simulink model "cic_dec3_4inputs_model"  (Simulink 7.4)
settings: Solver=ode45  StartTime=0.0  StopTime=10.0  RelTol=1e-3
libraries: xbsIndex_r4 x76
settings Model: Creator=chenhong  LastModifiedBy=chenhong

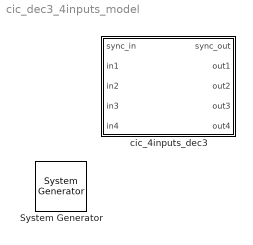
== system cic_dec3_4inputs_model ==
  " System Generator" : xbsIndex_r4/ System Generator  Tag=genX  SystemSampleTime=-1  xilinxfamily=Virtex6  part=xc6vsx315t  speed=-3  package=ff1156  synthesis_tool=XST  clock_wrapper=Clock Enables  directory=./netlist  testbench=off  simulink_period=1  sysclk_period=10  dcm_input_clock_period=10  incr_netlist=off  trim_vbits=Everywhere in SubSystem  dbl_ovrd=According to Block Masks  core_generation=According to Block Masks  run_coregen=off  deprecated_control=off  eval_field=0  block_type=sysgen
      settings: block_version=11.4
  cic_4inputs_dec3 : Subsystem

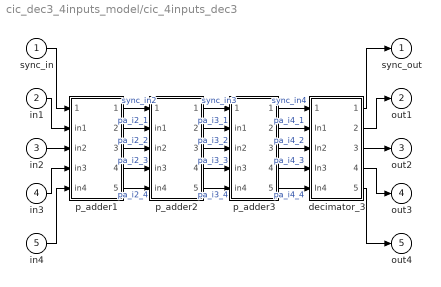
== system cic_dec3_4inputs_model/cic_4inputs_dec3 ==
  sync_in : Inport
  in1 : Inport  Port=2
  in2 : Inport  Port=3
  in3 : Inport  Port=4
  in4 : Inport  Port=5
  decimator_3 : Subsystem
  p_adder1 : Subsystem
  p_adder2 : Subsystem
  p_adder3 : Subsystem
  sync_out : Outport
  out1 : Outport  Port=2
  out2 : Outport  Port=3
  out3 : Outport  Port=4
  out4 : Outport  Port=5
  wires:
  decimator_3/4(Out3) -> out3/1
  decimator_3/2(Out1) -> out1/1
  p_adder3/5(out4) -> decimator_3/5(In4)  "pa_i4_4"
  p_adder3/3(out2) -> decimator_3/3(In2)  "pa_i4_2"
  p_adder3/1(sync_out) -> decimator_3/1(sync_in)  "sync_in4"
  p_adder2/5(out4) -> p_adder3/5(in4)  "pa_i3_4"
  p_adder2/3(out2) -> p_adder3/3(in2)  "pa_i3_2"
  p_adder2/1(sync_out) -> p_adder3/1(sync_in)  "sync_in3"
  p_adder1/5(out4) -> p_adder2/5(in4)  "pa_i2_4"
  p_adder1/3(out2) -> p_adder2/3(in2)  "pa_i2_2"
  p_adder1/1(sync_out) -> p_adder2/1(sync_in)  "sync_in2"
  in4/1 -> p_adder1/5(in4)
  in2/1 -> p_adder1/3(in2)
  sync_in/1 -> p_adder1/1(sync_in)
  in1/1 -> p_adder1/2(in1)
  in3/1 -> p_adder1/4(in3)
  p_adder1/2(out1) -> p_adder2/2(in1)  "pa_i2_1"
  p_adder1/4(out3) -> p_adder2/4(in3)  "pa_i2_3"
  p_adder2/2(out1) -> p_adder3/2(in1)  "pa_i3_1"
  p_adder2/4(out3) -> p_adder3/4(in3)  "pa_i3_3"
  p_adder3/2(out1) -> decimator_3/2(In1)  "pa_i4_1"
  p_adder3/4(out3) -> decimator_3/4(In3)  "pa_i4_3"
  decimator_3/1(sync_out) -> sync_out/1
  decimator_3/3(Out2) -> out2/1
  decimator_3/5(Out4) -> out4/1

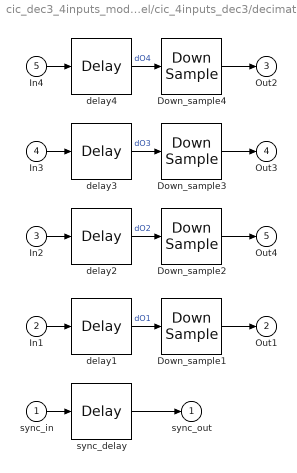
== system cic_dec3_4inputs_model/cic_4inputs_dec3/decimator_3 ==
  sync_in : Inport
  In1 : Inport  Port=2
  In2 : Inport  Port=3
  In3 : Inport  Port=4
  In4 : Inport  Port=5
  Down_sample{1..4} (4 alike) : xbsIndex_r4/Down Sample  sample_ratio=3  sample_phase="Last Value of Frame  (most efficient)"  en=off  latency=1  dbl_ovrd=off  block_type=dsamp
      settings: block_version=11.4
  delay1 : xbsIndex_r4/Delay  en=off  latency=2  dbl_ovrd=off  reg_retiming=off  block_type=delay
      settings: block_version=11.4
  delay2 : xbsIndex_r4/Delay  en=off  latency=0  dbl_ovrd=off  reg_retiming=off  block_type=delay
      settings: block_version=11.4
  delay3 : xbsIndex_r4/Delay  en=off  latency=1  dbl_ovrd=off  reg_retiming=off  block_type=delay
      settings: block_version=11.4
  delay4 : xbsIndex_r4/Delay  en=off  latency=2  dbl_ovrd=off  reg_retiming=off  block_type=delay
      settings: block_version=11.4
  sync_delay : xbsIndex_r4/Delay  en=off  latency=1  dbl_ovrd=off  reg_retiming=off  block_type=delay
      settings: block_version=11.4
  sync_out : Outport
  Out1 : Outport  Port=2
  Out2 : Outport  Port=3
  Out3 : Outport  Port=4
  Out4 : Outport  Port=5
  wires:
  sync_in/1 -> sync_delay/1
  Down_sample4/1 -> Out2/1
  delay3/1 -> Down_sample3/1  "dO3"
  In3/1 -> delay3/1
  Down_sample2/1 -> Out4/1
  delay1/1 -> Down_sample1/1  "dO1"
  In1/1 -> delay1/1
  Down_sample1/1 -> Out1/1
  In2/1 -> delay2/1
  delay2/1 -> Down_sample2/1  "dO2"
  Down_sample3/1 -> Out3/1
  In4/1 -> delay4/1
  delay4/1 -> Down_sample4/1  "dO4"
  sync_delay/1 -> sync_out/1

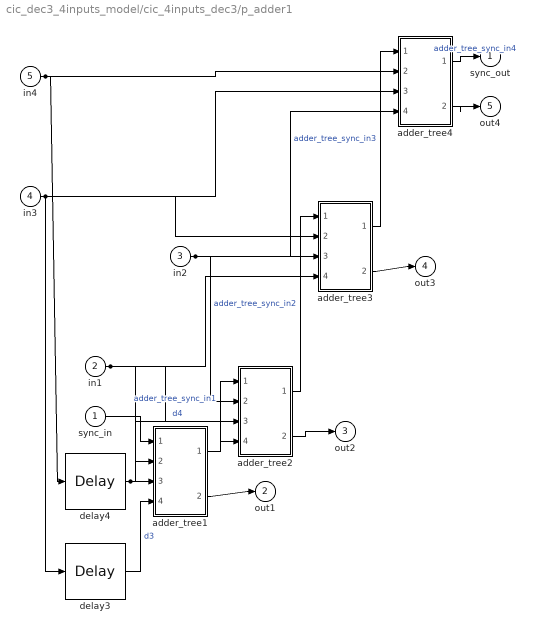
== system cic_dec3_4inputs_model/cic_4inputs_dec3/p_adder1 ==
  sync_in : Inport
  in1 : Inport  Port=2
  in2 : Inport  Port=3
  in3 : Inport  Port=4
  in4 : Inport  Port=5
  adder_tree1 : Subsystem
  adder_tree2 : Subsystem
  adder_tree3 : Subsystem
  adder_tree4 : Subsystem
  delay3 : xbsIndex_r4/Delay  en=off  latency=1  dbl_ovrd=off  reg_retiming=off  block_type=delay
      settings: block_version=11.4
  delay4 : xbsIndex_r4/Delay  en=off  latency=1  dbl_ovrd=off  reg_retiming=off  block_type=delay
      settings: block_version=11.4
  sync_out : Outport
  out1 : Outport  Port=2
  out2 : Outport  Port=3
  out3 : Outport  Port=4
  out4 : Outport  Port=5
  wires:
  in1/1 -> adder_tree2/3(din_2), adder_tree1/2(din_1), adder_tree3/4(din_3)
  delay4/1 -> adder_tree1/3(din_2), adder_tree2/4(din_3)  "d4"
  in3/1 -> adder_tree4/3(din_2), delay3/1, adder_tree3/2(din_1)
  in2/1 -> adder_tree3/3(din_2), adder_tree2/2(din_1), adder_tree4/4(din_3)
  in4/1 -> delay4/1, adder_tree4/2(din_1)
  adder_tree4/1(sync_out) -> sync_out/1  "adder_tree_sync_in4"
  adder_tree4/2(dout) -> out4/1
  adder_tree3/1(sync_out) -> adder_tree4/1(sync)  "adder_tree_sync_in3"
  adder_tree3/2(dout) -> out3/1
  adder_tree2/1(sync_out) -> adder_tree3/1(sync)  "adder_tree_sync_in2"
  adder_tree2/2(dout) -> out2/1
  adder_tree1/1(sync_out) -> adder_tree2/1(sync)  "adder_tree_sync_in1"
  adder_tree1/2(dout) -> out1/1
  sync_in/1 -> adder_tree1/1(sync)
  delay3/1 -> adder_tree1/4(din_3)  "d3"

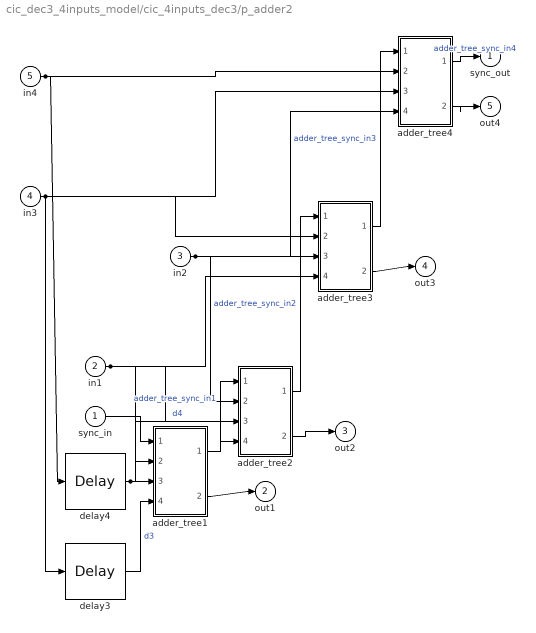
== system cic_dec3_4inputs_model/cic_4inputs_dec3/p_adder2 ==
  sync_in : Inport
  in1 : Inport  Port=2
  in2 : Inport  Port=3
  in3 : Inport  Port=4
  in4 : Inport  Port=5
  adder_tree1 : Subsystem
  adder_tree2 : Subsystem
  adder_tree3 : Subsystem
  adder_tree4 : Subsystem
  delay3 : xbsIndex_r4/Delay  en=off  latency=1  dbl_ovrd=off  reg_retiming=off  block_type=delay
      settings: block_version=11.4
  delay4 : xbsIndex_r4/Delay  en=off  latency=1  dbl_ovrd=off  reg_retiming=off  block_type=delay
      settings: block_version=11.4
  sync_out : Outport
  out1 : Outport  Port=2
  out2 : Outport  Port=3
  out3 : Outport  Port=4
  out4 : Outport  Port=5
  wires:
  in1/1 -> adder_tree2/3(din_2), adder_tree1/2(din_1), adder_tree3/4(din_3)
  delay4/1 -> adder_tree1/3(din_2), adder_tree2/4(din_3)  "d4"
  in3/1 -> adder_tree4/3(din_2), delay3/1, adder_tree3/2(din_1)
  in2/1 -> adder_tree3/3(din_2), adder_tree2/2(din_1), adder_tree4/4(din_3)
  in4/1 -> delay4/1, adder_tree4/2(din_1)
  adder_tree4/1(sync_out) -> sync_out/1  "adder_tree_sync_in4"
  adder_tree4/2(dout) -> out4/1
  adder_tree3/1(sync_out) -> adder_tree4/1(sync)  "adder_tree_sync_in3"
  adder_tree3/2(dout) -> out3/1
  adder_tree2/1(sync_out) -> adder_tree3/1(sync)  "adder_tree_sync_in2"
  adder_tree2/2(dout) -> out2/1
  adder_tree1/1(sync_out) -> adder_tree2/1(sync)  "adder_tree_sync_in1"
  adder_tree1/2(dout) -> out1/1
  sync_in/1 -> adder_tree1/1(sync)
  delay3/1 -> adder_tree1/4(din_3)  "d3"

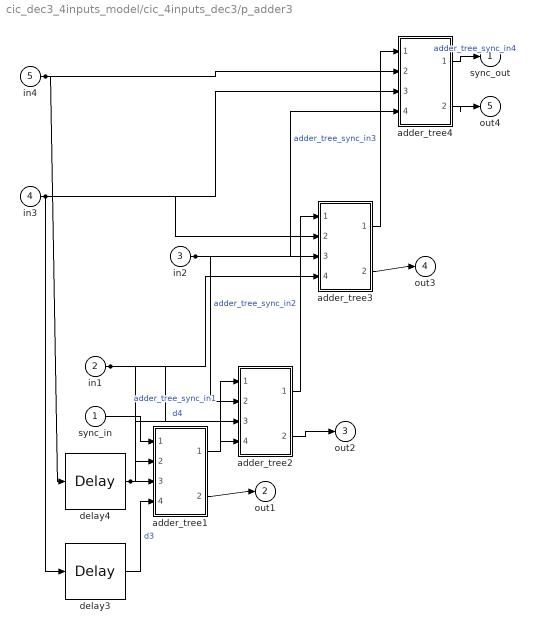
== system cic_dec3_4inputs_model/cic_4inputs_dec3/p_adder3 ==
  sync_in : Inport
  in1 : Inport  Port=2
  in2 : Inport  Port=3
  in3 : Inport  Port=4
  in4 : Inport  Port=5
  adder_tree1 : Subsystem
  adder_tree2 : Subsystem
  adder_tree3 : Subsystem
  adder_tree4 : Subsystem
  delay3 : xbsIndex_r4/Delay  en=off  latency=1  dbl_ovrd=off  reg_retiming=off  block_type=delay
      settings: block_version=11.4
  delay4 : xbsIndex_r4/Delay  en=off  latency=1  dbl_ovrd=off  reg_retiming=off  block_type=delay
      settings: block_version=11.4
  sync_out : Outport
  out1 : Outport  Port=2
  out2 : Outport  Port=3
  out3 : Outport  Port=4
  out4 : Outport  Port=5
  wires:
  in1/1 -> adder_tree2/3(din_2), adder_tree1/2(din_1), adder_tree3/4(din_3)
  delay4/1 -> adder_tree1/3(din_2), adder_tree2/4(din_3)  "d4"
  in3/1 -> adder_tree4/3(din_2), delay3/1, adder_tree3/2(din_1)
  in2/1 -> adder_tree3/3(din_2), adder_tree2/2(din_1), adder_tree4/4(din_3)
  in4/1 -> delay4/1, adder_tree4/2(din_1)
  adder_tree4/1(sync_out) -> sync_out/1  "adder_tree_sync_in4"
  adder_tree4/2(dout) -> out4/1
  adder_tree3/1(sync_out) -> adder_tree4/1(sync)  "adder_tree_sync_in3"
  adder_tree3/2(dout) -> out3/1
  adder_tree2/1(sync_out) -> adder_tree3/1(sync)  "adder_tree_sync_in2"
  adder_tree2/2(dout) -> out2/1
  adder_tree1/1(sync_out) -> adder_tree2/1(sync)  "adder_tree_sync_in1"
  adder_tree1/2(dout) -> out1/1
  sync_in/1 -> adder_tree1/1(sync)
  delay3/1 -> adder_tree1/4(din_3)  "d3"

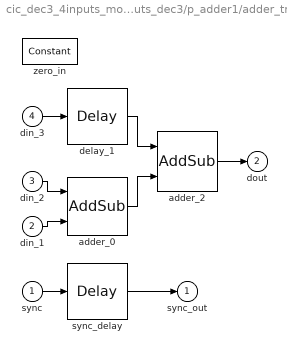
== system cic_dec3_4inputs_model/cic_4inputs_dec3/p_adder1/adder_tree1 ==
  sync : Inport
  din_1 : Inport  Port=2
  din_2 : Inport  Port=3
  din_3 : Inport  Port=4
  adder_0 : xbsIndex_r4/AddSub  mode=Addition  use_carryin=off  use_carryout=off  en=off  latency=1  precision=Full  arith_type=Unsigned  n_bits=16  bin_pt=14  quantization="Round  (unbiased: +/- Inf)"  overflow=Saturate  dbl_ovrd=off  use_behavioral_HDL=on  hw_selection=Fabric  pipelined=off  block_type=addsub
  adder_2 : xbsIndex_r4/AddSub  mode=Addition  use_carryin=off  use_carryout=off  en=off  latency=1  precision=Full  arith_type=Unsigned  n_bits=16  bin_pt=14  quantization="Round  (unbiased: +/- Inf)"  overflow=Saturate  dbl_ovrd=off  use_behavioral_HDL=on  hw_selection=Fabric  pipelined=off  block_type=addsub
  delay_1 : xbsIndex_r4/Delay  en=off  latency=1  dbl_ovrd=off  reg_retiming=off  block_type=delay
      settings: block_version=11.4
  sync_delay : xbsIndex_r4/Delay  en=off  latency=2  dbl_ovrd=off  reg_retiming=off  block_type=delay
      settings: block_version=11.4
  zero_in : xbsIndex_r4/Constant  arith_type=Unsigned  const=0  n_bits=18  bin_pt=17  explicit_period=off  period=1  equ=P=C  opselect=C  inp2=PCIN>>17  opr=+  inp1=P  carry=CIN  dbl_ovrd=off  block_type=constant
      settings: block_version=11.4
  sync_out : Outport
  dout : Outport  Port=2
  wires:
  adder_0/1 -> adder_2/2
  din_2/1 -> adder_0/1
  sync/1 -> sync_delay/1
  sync_delay/1 -> sync_out/1
  din_1/1 -> adder_0/2
  din_3/1 -> delay_1/1
  delay_1/1 -> adder_2/1
  adder_2/1 -> dout/1

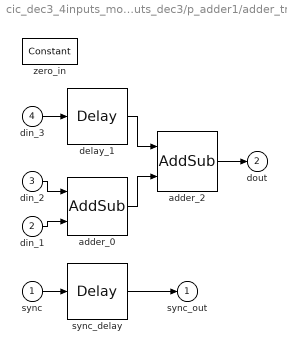
== system cic_dec3_4inputs_model/cic_4inputs_dec3/p_adder1/adder_tree2 ==
  sync : Inport
  din_1 : Inport  Port=2
  din_2 : Inport  Port=3
  din_3 : Inport  Port=4
  adder_0 : xbsIndex_r4/AddSub  mode=Addition  use_carryin=off  use_carryout=off  en=off  latency=1  precision=Full  arith_type=Unsigned  n_bits=16  bin_pt=14  quantization="Round  (unbiased: +/- Inf)"  overflow=Saturate  dbl_ovrd=off  use_behavioral_HDL=on  hw_selection=Fabric  pipelined=off  block_type=addsub
  adder_2 : xbsIndex_r4/AddSub  mode=Addition  use_carryin=off  use_carryout=off  en=off  latency=1  precision=Full  arith_type=Unsigned  n_bits=16  bin_pt=14  quantization="Round  (unbiased: +/- Inf)"  overflow=Saturate  dbl_ovrd=off  use_behavioral_HDL=on  hw_selection=Fabric  pipelined=off  block_type=addsub
  delay_1 : xbsIndex_r4/Delay  en=off  latency=1  dbl_ovrd=off  reg_retiming=off  block_type=delay
      settings: block_version=11.4
  sync_delay : xbsIndex_r4/Delay  en=off  latency=2  dbl_ovrd=off  reg_retiming=off  block_type=delay
      settings: block_version=11.4
  zero_in : xbsIndex_r4/Constant  arith_type=Unsigned  const=0  n_bits=18  bin_pt=17  explicit_period=off  period=1  equ=P=C  opselect=C  inp2=PCIN>>17  opr=+  inp1=P  carry=CIN  dbl_ovrd=off  block_type=constant
      settings: block_version=11.4
  sync_out : Outport
  dout : Outport  Port=2
  wires:
  adder_0/1 -> adder_2/2
  din_2/1 -> adder_0/1
  sync/1 -> sync_delay/1
  sync_delay/1 -> sync_out/1
  din_1/1 -> adder_0/2
  din_3/1 -> delay_1/1
  delay_1/1 -> adder_2/1
  adder_2/1 -> dout/1

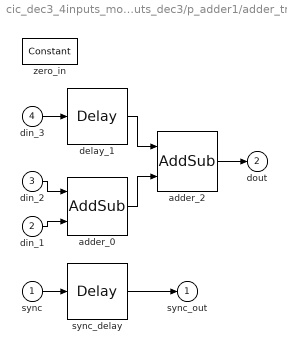
== system cic_dec3_4inputs_model/cic_4inputs_dec3/p_adder1/adder_tree3 ==
  sync : Inport
  din_1 : Inport  Port=2
  din_2 : Inport  Port=3
  din_3 : Inport  Port=4
  adder_0 : xbsIndex_r4/AddSub  mode=Addition  use_carryin=off  use_carryout=off  en=off  latency=1  precision=Full  arith_type=Unsigned  n_bits=16  bin_pt=14  quantization="Round  (unbiased: +/- Inf)"  overflow=Saturate  dbl_ovrd=off  use_behavioral_HDL=on  hw_selection=Fabric  pipelined=off  block_type=addsub
  adder_2 : xbsIndex_r4/AddSub  mode=Addition  use_carryin=off  use_carryout=off  en=off  latency=1  precision=Full  arith_type=Unsigned  n_bits=16  bin_pt=14  quantization="Round  (unbiased: +/- Inf)"  overflow=Saturate  dbl_ovrd=off  use_behavioral_HDL=on  hw_selection=Fabric  pipelined=off  block_type=addsub
  delay_1 : xbsIndex_r4/Delay  en=off  latency=1  dbl_ovrd=off  reg_retiming=off  block_type=delay
      settings: block_version=11.4
  sync_delay : xbsIndex_r4/Delay  en=off  latency=2  dbl_ovrd=off  reg_retiming=off  block_type=delay
      settings: block_version=11.4
  zero_in : xbsIndex_r4/Constant  arith_type=Unsigned  const=0  n_bits=18  bin_pt=17  explicit_period=off  period=1  equ=P=C  opselect=C  inp2=PCIN>>17  opr=+  inp1=P  carry=CIN  dbl_ovrd=off  block_type=constant
      settings: block_version=11.4
  sync_out : Outport
  dout : Outport  Port=2
  wires:
  adder_0/1 -> adder_2/2
  din_2/1 -> adder_0/1
  sync/1 -> sync_delay/1
  sync_delay/1 -> sync_out/1
  din_1/1 -> adder_0/2
  din_3/1 -> delay_1/1
  delay_1/1 -> adder_2/1
  adder_2/1 -> dout/1

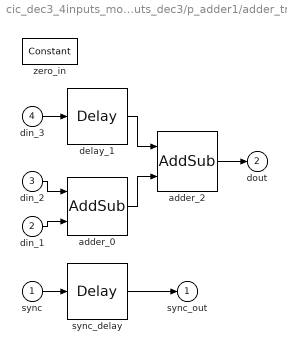
== system cic_dec3_4inputs_model/cic_4inputs_dec3/p_adder1/adder_tree4 ==
  sync : Inport
  din_1 : Inport  Port=2
  din_2 : Inport  Port=3
  din_3 : Inport  Port=4
  adder_0 : xbsIndex_r4/AddSub  mode=Addition  use_carryin=off  use_carryout=off  en=off  latency=1  precision=Full  arith_type=Unsigned  n_bits=16  bin_pt=14  quantization="Round  (unbiased: +/- Inf)"  overflow=Saturate  dbl_ovrd=off  use_behavioral_HDL=on  hw_selection=Fabric  pipelined=off  block_type=addsub
  adder_2 : xbsIndex_r4/AddSub  mode=Addition  use_carryin=off  use_carryout=off  en=off  latency=1  precision=Full  arith_type=Unsigned  n_bits=16  bin_pt=14  quantization="Round  (unbiased: +/- Inf)"  overflow=Saturate  dbl_ovrd=off  use_behavioral_HDL=on  hw_selection=Fabric  pipelined=off  block_type=addsub
  delay_1 : xbsIndex_r4/Delay  en=off  latency=1  dbl_ovrd=off  reg_retiming=off  block_type=delay
      settings: block_version=11.4
  sync_delay : xbsIndex_r4/Delay  en=off  latency=2  dbl_ovrd=off  reg_retiming=off  block_type=delay
      settings: block_version=11.4
  zero_in : xbsIndex_r4/Constant  arith_type=Unsigned  const=0  n_bits=18  bin_pt=17  explicit_period=off  period=1  equ=P=C  opselect=C  inp2=PCIN>>17  opr=+  inp1=P  carry=CIN  dbl_ovrd=off  block_type=constant
      settings: block_version=11.4
  sync_out : Outport
  dout : Outport  Port=2
  wires:
  adder_0/1 -> adder_2/2
  din_2/1 -> adder_0/1
  sync/1 -> sync_delay/1
  sync_delay/1 -> sync_out/1
  din_1/1 -> adder_0/2
  din_3/1 -> delay_1/1
  delay_1/1 -> adder_2/1
  adder_2/1 -> dout/1

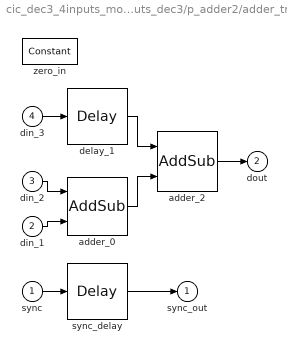
== system cic_dec3_4inputs_model/cic_4inputs_dec3/p_adder2/adder_tree1 ==
  sync : Inport
  din_1 : Inport  Port=2
  din_2 : Inport  Port=3
  din_3 : Inport  Port=4
  adder_0 : xbsIndex_r4/AddSub  mode=Addition  use_carryin=off  use_carryout=off  en=off  latency=1  precision=Full  arith_type=Unsigned  n_bits=16  bin_pt=14  quantization="Round  (unbiased: +/- Inf)"  overflow=Saturate  dbl_ovrd=off  use_behavioral_HDL=on  hw_selection=Fabric  pipelined=off  block_type=addsub
  adder_2 : xbsIndex_r4/AddSub  mode=Addition  use_carryin=off  use_carryout=off  en=off  latency=1  precision=Full  arith_type=Unsigned  n_bits=16  bin_pt=14  quantization="Round  (unbiased: +/- Inf)"  overflow=Saturate  dbl_ovrd=off  use_behavioral_HDL=on  hw_selection=Fabric  pipelined=off  block_type=addsub
  delay_1 : xbsIndex_r4/Delay  en=off  latency=1  dbl_ovrd=off  reg_retiming=off  block_type=delay
      settings: block_version=11.4
  sync_delay : xbsIndex_r4/Delay  en=off  latency=2  dbl_ovrd=off  reg_retiming=off  block_type=delay
      settings: block_version=11.4
  zero_in : xbsIndex_r4/Constant  arith_type=Unsigned  const=0  n_bits=18  bin_pt=17  explicit_period=off  period=1  equ=P=C  opselect=C  inp2=PCIN>>17  opr=+  inp1=P  carry=CIN  dbl_ovrd=off  block_type=constant
      settings: block_version=11.4
  sync_out : Outport
  dout : Outport  Port=2
  wires:
  adder_0/1 -> adder_2/2
  din_2/1 -> adder_0/1
  sync/1 -> sync_delay/1
  sync_delay/1 -> sync_out/1
  din_1/1 -> adder_0/2
  din_3/1 -> delay_1/1
  delay_1/1 -> adder_2/1
  adder_2/1 -> dout/1

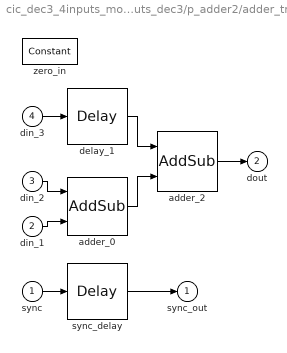
== system cic_dec3_4inputs_model/cic_4inputs_dec3/p_adder2/adder_tree2 ==
  sync : Inport
  din_1 : Inport  Port=2
  din_2 : Inport  Port=3
  din_3 : Inport  Port=4
  adder_0 : xbsIndex_r4/AddSub  mode=Addition  use_carryin=off  use_carryout=off  en=off  latency=1  precision=Full  arith_type=Unsigned  n_bits=16  bin_pt=14  quantization="Round  (unbiased: +/- Inf)"  overflow=Saturate  dbl_ovrd=off  use_behavioral_HDL=on  hw_selection=Fabric  pipelined=off  block_type=addsub
  adder_2 : xbsIndex_r4/AddSub  mode=Addition  use_carryin=off  use_carryout=off  en=off  latency=1  precision=Full  arith_type=Unsigned  n_bits=16  bin_pt=14  quantization="Round  (unbiased: +/- Inf)"  overflow=Saturate  dbl_ovrd=off  use_behavioral_HDL=on  hw_selection=Fabric  pipelined=off  block_type=addsub
  delay_1 : xbsIndex_r4/Delay  en=off  latency=1  dbl_ovrd=off  reg_retiming=off  block_type=delay
      settings: block_version=11.4
  sync_delay : xbsIndex_r4/Delay  en=off  latency=2  dbl_ovrd=off  reg_retiming=off  block_type=delay
      settings: block_version=11.4
  zero_in : xbsIndex_r4/Constant  arith_type=Unsigned  const=0  n_bits=18  bin_pt=17  explicit_period=off  period=1  equ=P=C  opselect=C  inp2=PCIN>>17  opr=+  inp1=P  carry=CIN  dbl_ovrd=off  block_type=constant
      settings: block_version=11.4
  sync_out : Outport
  dout : Outport  Port=2
  wires:
  adder_0/1 -> adder_2/2
  din_2/1 -> adder_0/1
  sync/1 -> sync_delay/1
  sync_delay/1 -> sync_out/1
  din_1/1 -> adder_0/2
  din_3/1 -> delay_1/1
  delay_1/1 -> adder_2/1
  adder_2/1 -> dout/1

== system cic_dec3_4inputs_model/cic_4inputs_dec3/p_adder2/adder_tree3 ==
  sync : Inport
  din_1 : Inport  Port=2
  din_2 : Inport  Port=3
  din_3 : Inport  Port=4
  adder_0 : xbsIndex_r4/AddSub  mode=Addition  use_carryin=off  use_carryout=off  en=off  latency=1  precision=Full  arith_type=Unsigned  n_bits=16  bin_pt=14  quantization="Round  (unbiased: +/- Inf)"  overflow=Saturate  dbl_ovrd=off  use_behavioral_HDL=on  hw_selection=Fabric  pipelined=off  block_type=addsub
  adder_2 : xbsIndex_r4/AddSub  mode=Addition  use_carryin=off  use_carryout=off  en=off  latency=1  precision=Full  arith_type=Unsigned  n_bits=16  bin_pt=14  quantization="Round  (unbiased: +/- Inf)"  overflow=Saturate  dbl_ovrd=off  use_behavioral_HDL=on  hw_selection=Fabric  pipelined=off  block_type=addsub
  delay_1 : xbsIndex_r4/Delay  en=off  latency=1  dbl_ovrd=off  reg_retiming=off  block_type=delay
      settings: block_version=11.4
  sync_delay : xbsIndex_r4/Delay  en=off  latency=2  dbl_ovrd=off  reg_retiming=off  block_type=delay
      settings: block_version=11.4
  zero_in : xbsIndex_r4/Constant  arith_type=Unsigned  const=0  n_bits=18  bin_pt=17  explicit_period=off  period=1  equ=P=C  opselect=C  inp2=PCIN>>17  opr=+  inp1=P  carry=CIN  dbl_ovrd=off  block_type=constant
      settings: block_version=11.4
  sync_out : Outport
  dout : Outport  Port=2
  wires:
  adder_0/1 -> adder_2/2
  din_2/1 -> adder_0/1
  sync/1 -> sync_delay/1
  sync_delay/1 -> sync_out/1
  din_1/1 -> adder_0/2
  din_3/1 -> delay_1/1
  delay_1/1 -> adder_2/1
  adder_2/1 -> dout/1

== system cic_dec3_4inputs_model/cic_4inputs_dec3/p_adder2/adder_tree4 ==
  sync : Inport
  din_1 : Inport  Port=2
  din_2 : Inport  Port=3
  din_3 : Inport  Port=4
  adder_0 : xbsIndex_r4/AddSub  mode=Addition  use_carryin=off  use_carryout=off  en=off  latency=1  precision=Full  arith_type=Unsigned  n_bits=16  bin_pt=14  quantization="Round  (unbiased: +/- Inf)"  overflow=Saturate  dbl_ovrd=off  use_behavioral_HDL=on  hw_selection=Fabric  pipelined=off  block_type=addsub
  adder_2 : xbsIndex_r4/AddSub  mode=Addition  use_carryin=off  use_carryout=off  en=off  latency=1  precision=Full  arith_type=Unsigned  n_bits=16  bin_pt=14  quantization="Round  (unbiased: +/- Inf)"  overflow=Saturate  dbl_ovrd=off  use_behavioral_HDL=on  hw_selection=Fabric  pipelined=off  block_type=addsub
  delay_1 : xbsIndex_r4/Delay  en=off  latency=1  dbl_ovrd=off  reg_retiming=off  block_type=delay
      settings: block_version=11.4
  sync_delay : xbsIndex_r4/Delay  en=off  latency=2  dbl_ovrd=off  reg_retiming=off  block_type=delay
      settings: block_version=11.4
  zero_in : xbsIndex_r4/Constant  arith_type=Unsigned  const=0  n_bits=18  bin_pt=17  explicit_period=off  period=1  equ=P=C  opselect=C  inp2=PCIN>>17  opr=+  inp1=P  carry=CIN  dbl_ovrd=off  block_type=constant
      settings: block_version=11.4
  sync_out : Outport
  dout : Outport  Port=2
  wires:
  adder_0/1 -> adder_2/2
  din_2/1 -> adder_0/1
  sync/1 -> sync_delay/1
  sync_delay/1 -> sync_out/1
  din_1/1 -> adder_0/2
  din_3/1 -> delay_1/1
  delay_1/1 -> adder_2/1
  adder_2/1 -> dout/1

== system cic_dec3_4inputs_model/cic_4inputs_dec3/p_adder3/adder_tree1 ==
  sync : Inport
  din_1 : Inport  Port=2
  din_2 : Inport  Port=3
  din_3 : Inport  Port=4
  adder_0 : xbsIndex_r4/AddSub  mode=Addition  use_carryin=off  use_carryout=off  en=off  latency=1  precision=Full  arith_type=Unsigned  n_bits=16  bin_pt=14  quantization="Round  (unbiased: +/- Inf)"  overflow=Saturate  dbl_ovrd=off  use_behavioral_HDL=on  hw_selection=Fabric  pipelined=off  block_type=addsub
  adder_2 : xbsIndex_r4/AddSub  mode=Addition  use_carryin=off  use_carryout=off  en=off  latency=1  precision=Full  arith_type=Unsigned  n_bits=16  bin_pt=14  quantization="Round  (unbiased: +/- Inf)"  overflow=Saturate  dbl_ovrd=off  use_behavioral_HDL=on  hw_selection=Fabric  pipelined=off  block_type=addsub
  delay_1 : xbsIndex_r4/Delay  en=off  latency=1  dbl_ovrd=off  reg_retiming=off  block_type=delay
      settings: block_version=11.4
  sync_delay : xbsIndex_r4/Delay  en=off  latency=2  dbl_ovrd=off  reg_retiming=off  block_type=delay
      settings: block_version=11.4
  zero_in : xbsIndex_r4/Constant  arith_type=Unsigned  const=0  n_bits=18  bin_pt=17  explicit_period=off  period=1  equ=P=C  opselect=C  inp2=PCIN>>17  opr=+  inp1=P  carry=CIN  dbl_ovrd=off  block_type=constant
      settings: block_version=11.4
  sync_out : Outport
  dout : Outport  Port=2
  wires:
  adder_0/1 -> adder_2/2
  din_2/1 -> adder_0/1
  sync/1 -> sync_delay/1
  sync_delay/1 -> sync_out/1
  din_1/1 -> adder_0/2
  din_3/1 -> delay_1/1
  delay_1/1 -> adder_2/1
  adder_2/1 -> dout/1

== system cic_dec3_4inputs_model/cic_4inputs_dec3/p_adder3/adder_tree2 ==
  sync : Inport
  din_1 : Inport  Port=2
  din_2 : Inport  Port=3
  din_3 : Inport  Port=4
  adder_0 : xbsIndex_r4/AddSub  mode=Addition  use_carryin=off  use_carryout=off  en=off  latency=1  precision=Full  arith_type=Unsigned  n_bits=16  bin_pt=14  quantization="Round  (unbiased: +/- Inf)"  overflow=Saturate  dbl_ovrd=off  use_behavioral_HDL=on  hw_selection=Fabric  pipelined=off  block_type=addsub
  adder_2 : xbsIndex_r4/AddSub  mode=Addition  use_carryin=off  use_carryout=off  en=off  latency=1  precision=Full  arith_type=Unsigned  n_bits=16  bin_pt=14  quantization="Round  (unbiased: +/- Inf)"  overflow=Saturate  dbl_ovrd=off  use_behavioral_HDL=on  hw_selection=Fabric  pipelined=off  block_type=addsub
  delay_1 : xbsIndex_r4/Delay  en=off  latency=1  dbl_ovrd=off  reg_retiming=off  block_type=delay
      settings: block_version=11.4
  sync_delay : xbsIndex_r4/Delay  en=off  latency=2  dbl_ovrd=off  reg_retiming=off  block_type=delay
      settings: block_version=11.4
  zero_in : xbsIndex_r4/Constant  arith_type=Unsigned  const=0  n_bits=18  bin_pt=17  explicit_period=off  period=1  equ=P=C  opselect=C  inp2=PCIN>>17  opr=+  inp1=P  carry=CIN  dbl_ovrd=off  block_type=constant
      settings: block_version=11.4
  sync_out : Outport
  dout : Outport  Port=2
  wires:
  adder_0/1 -> adder_2/2
  din_2/1 -> adder_0/1
  sync/1 -> sync_delay/1
  sync_delay/1 -> sync_out/1
  din_1/1 -> adder_0/2
  din_3/1 -> delay_1/1
  delay_1/1 -> adder_2/1
  adder_2/1 -> dout/1

== system cic_dec3_4inputs_model/cic_4inputs_dec3/p_adder3/adder_tree3 ==
  sync : Inport
  din_1 : Inport  Port=2
  din_2 : Inport  Port=3
  din_3 : Inport  Port=4
  adder_0 : xbsIndex_r4/AddSub  mode=Addition  use_carryin=off  use_carryout=off  en=off  latency=1  precision=Full  arith_type=Unsigned  n_bits=16  bin_pt=14  quantization="Round  (unbiased: +/- Inf)"  overflow=Saturate  dbl_ovrd=off  use_behavioral_HDL=on  hw_selection=Fabric  pipelined=off  block_type=addsub
  adder_2 : xbsIndex_r4/AddSub  mode=Addition  use_carryin=off  use_carryout=off  en=off  latency=1  precision=Full  arith_type=Unsigned  n_bits=16  bin_pt=14  quantization="Round  (unbiased: +/- Inf)"  overflow=Saturate  dbl_ovrd=off  use_behavioral_HDL=on  hw_selection=Fabric  pipelined=off  block_type=addsub
  delay_1 : xbsIndex_r4/Delay  en=off  latency=1  dbl_ovrd=off  reg_retiming=off  block_type=delay
      settings: block_version=11.4
  sync_delay : xbsIndex_r4/Delay  en=off  latency=2  dbl_ovrd=off  reg_retiming=off  block_type=delay
      settings: block_version=11.4
  zero_in : xbsIndex_r4/Constant  arith_type=Unsigned  const=0  n_bits=18  bin_pt=17  explicit_period=off  period=1  equ=P=C  opselect=C  inp2=PCIN>>17  opr=+  inp1=P  carry=CIN  dbl_ovrd=off  block_type=constant
      settings: block_version=11.4
  sync_out : Outport
  dout : Outport  Port=2
  wires:
  adder_0/1 -> adder_2/2
  din_2/1 -> adder_0/1
  sync/1 -> sync_delay/1
  sync_delay/1 -> sync_out/1
  din_1/1 -> adder_0/2
  din_3/1 -> delay_1/1
  delay_1/1 -> adder_2/1
  adder_2/1 -> dout/1

== system cic_dec3_4inputs_model/cic_4inputs_dec3/p_adder3/adder_tree4 ==
  sync : Inport
  din_1 : Inport  Port=2
  din_2 : Inport  Port=3
  din_3 : Inport  Port=4
  adder_0 : xbsIndex_r4/AddSub  mode=Addition  use_carryin=off  use_carryout=off  en=off  latency=1  precision=Full  arith_type=Unsigned  n_bits=16  bin_pt=14  quantization="Round  (unbiased: +/- Inf)"  overflow=Saturate  dbl_ovrd=off  use_behavioral_HDL=on  hw_selection=Fabric  pipelined=off  block_type=addsub
  adder_2 : xbsIndex_r4/AddSub  mode=Addition  use_carryin=off  use_carryout=off  en=off  latency=1  precision=Full  arith_type=Unsigned  n_bits=16  bin_pt=14  quantization="Round  (unbiased: +/- Inf)"  overflow=Saturate  dbl_ovrd=off  use_behavioral_HDL=on  hw_selection=Fabric  pipelined=off  block_type=addsub
  delay_1 : xbsIndex_r4/Delay  en=off  latency=1  dbl_ovrd=off  reg_retiming=off  block_type=delay
      settings: block_version=11.4
  sync_delay : xbsIndex_r4/Delay  en=off  latency=2  dbl_ovrd=off  reg_retiming=off  block_type=delay
      settings: block_version=11.4
  zero_in : xbsIndex_r4/Constant  arith_type=Unsigned  const=0  n_bits=18  bin_pt=17  explicit_period=off  period=1  equ=P=C  opselect=C  inp2=PCIN>>17  opr=+  inp1=P  carry=CIN  dbl_ovrd=off  block_type=constant
      settings: block_version=11.4
  sync_out : Outport
  dout : Outport  Port=2
  wires:
  adder_0/1 -> adder_2/2
  din_2/1 -> adder_0/1
  sync/1 -> sync_delay/1
  sync_delay/1 -> sync_out/1
  din_1/1 -> adder_0/2
  din_3/1 -> delay_1/1
  delay_1/1 -> adder_2/1
  adder_2/1 -> dout/1
